simulink model "CS637Assignment1_3_1"  (R2022a)
settings: Solver=VariableStepAuto  StartTime=0.0  StopTime=1000.0  RelTol=1e-3
settings Model: Creator=kaush  LastModifiedBy=kaush

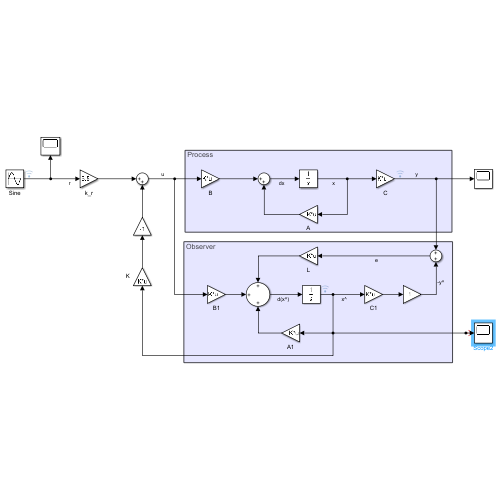
[thumbnail: Simulink's stored preview of the top-level diagram]
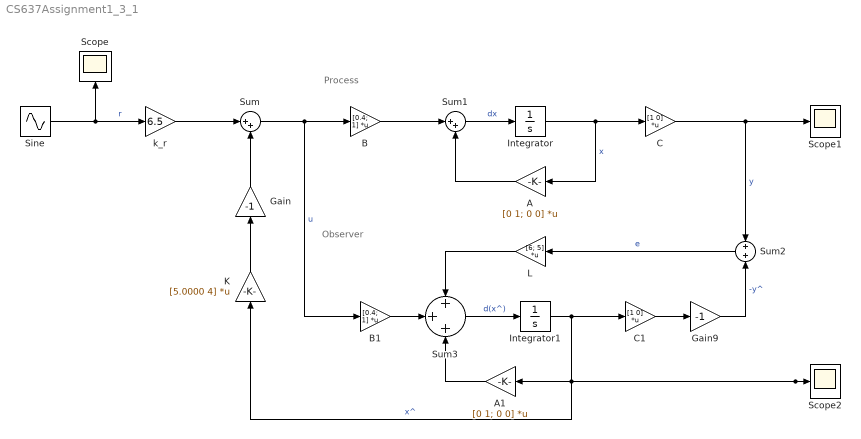
== system CS637Assignment1_3_1 ==
  note: Process
  note: Observer
  A : Gain  Gain=[0 1; 0 0]  Multiplication=Matrix(K*u)
  A1 : Gain  Gain=[0 1; 0 0]  Multiplication=Matrix(K*u)
  B : Gain  Gain=[0.4; 1]  Multiplication=Matrix(K*u)
  B1 : Gain  Gain=[0.4; 1]  Multiplication=Matrix(K*u)
  C : Gain  Gain=[1 0]  Multiplication=Matrix(K*u)
  C1 : Gain  Gain=[1 0]  Multiplication=Matrix(K*u)
  Gain : Gain  Gain=-1
  Gain9 : Gain  Gain=-1
  Integrator : Integrator
  Integrator1 : Integrator
  K : Gain  Gain=[5.0000 4]  Multiplication=Matrix(K*u)
  L : Gain  Gain=[6; 5]  Multiplication=Matrix(K*u)
  Scope : Scope
  Scope1 : Scope
  Scope2 : Scope
  Sine : Sin  SampleTime=0
  Sum : Sum  Inputs=|++
  Sum1 : Sum  Inputs=|++
  Sum2 : Sum
  Sum3 : Sum  Inputs=+++
  k_r : Gain  Gain=6.5
  wires:
  Sine/1 -> k_r/1, Scope/1  "r"
  k_r/1 -> Sum/1
  K/1 -> Gain/1
  Sum/1 -> B1/1, B/1  "u"
  B/1 -> Sum1/1
  Sum1/1 -> Integrator/1  "dx"
  A/1 -> Sum1/2
  Integrator/1 -> A/1, C/1  "x"
  C/1 -> Scope1/1, Sum2/1  "y"
  B1/1 -> Sum3/2
  Sum2/1 -> L/1  "e"
  Sum3/1 -> Integrator1/1  "d(x^)"
  A1/1 -> Sum3/3
  C1/1 -> Gain9/1
  Gain9/1 -> Sum2/2  "-y^"
  Integrator1/1 -> Scope2/1, K/1, A1/1, C1/1  "x^"
  L/1 -> Sum3/1
  Gain/1 -> Sum/2
